simulink model "untitled1"  (R2024a)
settings: Solver=VariableStepAuto  StartTime=0.0  StopTime=50  RelTol=1e-3
settings Model: Creator=ashis  LastModifiedBy=ashis

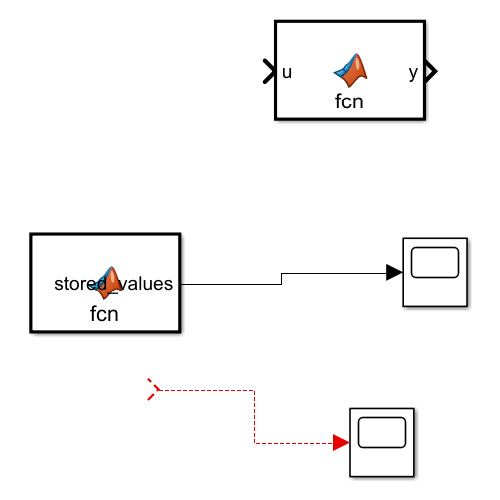
[thumbnail: Simulink's stored preview of the top-level diagram]
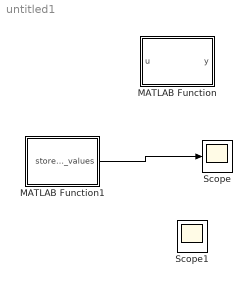
== system untitled1 ==
  MATLAB Function : MATLAB Function  TreatAsAtomicUnit=on
  MATLAB Function1 : MATLAB Function  TreatAsAtomicUnit=on
  Scope : Scope
  Scope1 : Scope
  wires:
  MATLAB Function1/1(stored_values) -> Scope/1
  ? -> Scope1/1

== matlab function untitled1/MATLAB Function ==
  data: u input; y output
function y = fcn(u)

y = u

== matlab function untitled1/MATLAB Function1 ==
  data: stored_values output
function stored_values = fcn()
    % Declare extrinsic functions
    coder.extrinsic('serialport');
    coder.extrinsic('readline');
    coder.extrinsic('split');
    coder.extrinsic('str2double');

    % Persistent variable to store the Arduino object
    persistent arduino;

    if isempty(arduino)
        % Initialize the serial port (only done once)
        arduino = serialport("COM2", 9600);
        
    end

    % Initialize stored_values as zeros
    
   var = readline(arduino) ;
   parts = split(var, ',');
   stored_values = zeros(4, 1);
    % Assign values to stored_values (assuming we want the first four values)
    for i = 1:4
        stored_values(i) = str2double(parts(i));
    end

end
